simulink model "sm_robot_run_4legs"  (R2022b)
settings: Solver=ode15s  StartTime=0.0  StopTime=2  MaxStep=0.01  RelTol=1e-3  AbsTol=1e-4  EnableMultiTasking=on
InitFcn:
  | d2r = pi/180;
  | r2d = 180/pi;
  | if (~exist('t_final'))
  |   sm_robot_run_4legs_param_def_load(bdroot)
  | end
undefined symbols (not defined in the file): body_width, bw, Extr_Data_LinkEndHole, Extr_Data_Mesh, J, l1, L_back, L_stance, M, N, T_cg, t_th, t_w, th2, th2_0, Trq_propulsive, u0, u_th, u_w, X, Y, Z
libraries: sm_lib x60, fl_lib x57, nesl_utility x26, ee_lib x4, sm_robot_run_4legs_lib x4, batteryecm_lib x1
(part 4 of 4)

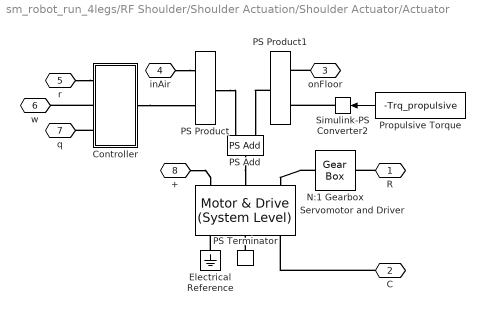
== system sm_robot_run_4legs/RF Shoulder/Shoulder Actuation/Shoulder Actuator/Actuator ==
  Controller : Subsystem
  Electrical Reference : fl_lib/Electrical/Electrical Elements/Electrical Reference
  N:1 Gearbox : fl_lib/Mechanical/Mechanisms/Gear Box  ratio=-N  t_in_specify=off  t_in_priority=None  t_in=0 N*m  t_in_nominal_specify=off  t_in_nominal_unit=N*m  t_in_nominal_value=1  t_out_specify=off  t_out_priority=None  t_out=0 N*m  t_out_nominal_specify=off  t_out_nominal_unit=N*m  t_out_nominal_value=1
  PS Add : fl_lib/Physical Signals/Functions/PS Add
  PS Product : fl_lib/Physical Signals/Functions/PS Product
  PS Product1 : fl_lib/Physical Signals/Functions/PS Product
  PS Terminator : fl_lib/Physical Signals/Sinks/PS Terminator
  Propulsive Torque : Constant  Value=-Trq_propulsive
  Servomotor and Driver : ee_lib/Electromechanical/Motor & Drive (System Level)  torque_speed_param=1  overtorque_param=ee.enum.electromech.overtorque.no  T_t="[  0.13 0.115 0.1 0 ]*5 N*m"  T_t_intermittent=[.36, .32, .28, 0] N*m  T_t_2D=[.09, .09, .09; .08, .08, .08; .07, .07, .07; 0, 0, 0] N*m  T_t_intermittent_2D=[.36, .36, .36; .32, .32, .32; .28, .28, .28; 0, 0, 0] N*m  w_t="[  0 2e+03 4e+03 4.1e3] rpm"  vdc_t=[6, 12, 24] V  torque_max=0.1 N*m  power_max=30 W  torque_max_intermittent=0.4 N*m  power_max_intermittent=120 W  time_overtorque=30 s  time_recover=60 s  Tc=0.01 s  losses_param=1  eff=100  w_eff=3.75e+3 rpm  T_eff=0.08 N*m  Piron=0 W  Pbase=0 W  w_eff_vec=[-8000 -4000 0 4000 8000] rpm  T_eff_vec=[0 0.03 0.06 0.09] N*m  v_eff_vec=[100, 250, 400] V  losses_mat=[1.49 1.67 2.21 3.10; 0.42 0.69 1.14 2.03; 0.06 0.24 0.78 1.68; 0.42 0.69 1.14 2.03; 1.49 1.67 2.21 3.10] W  efficiency_mat=[95 95 95 95; 95 95 95 95; 95 95 95 95; 95 95 95 95; 95 95 95 95]  losses_mat_3D=ones(5, 4, 3) W  efficiency_mat_3D=95 * ones(5, 4, 3)  Res=0.1 Ohm  enable_fault=simscape.enum.onoff.off  fault_condition=1  fault_threshold=0.5  J=0 g*cm^2  lam=0 N*m/(rad/s)  speed0=th1_dot_0*N rad/s  faulted_specify=off  faulted_priority=None  faulted=0  faulted_nominal_specify=off  faulted_nominal_unit=1  faulted_nominal_value=1  torqueLimitContinuous_specify=off  torqueLimitContinuous_priority=None  torqueLimitContinuous=0 N*m  torqueLimitContinuous_nominal_specify=off  torqueLimitContinuous_nominal_unit=N*m  torqueLimitContinuous_nominal_value=1  alpha=3.93e-3 1/K  Tmeas=25 degC  Tmeas2=125 degC  losses_mat_T2=[1.49, 1.74, 2.49, 3.74; .42, .67, 1.42, 2.67; .06, .31, 1.06, 2.31; .42, .67, 1.42, 2.67; 1.49, 1.74, 2.49, 3.74] W  efficiency_mat_T2=[95, 95, 95, 95; 95, 95, 95, 95; 95, 95, 95, 95; 95, 95, 95, 95; 95, 95, 95, 95]  losses_mat_3D_T2=ones(5, 4, 3) W  efficiency_mat_3D_T2=95 * ones(5, 4, 3)  thermal_mass=100 J/K  initial_temperature=25 degC
  Simulink-PS Converter2 : nesl_utility/Simulink-PS Converter  PhysicalDomain=network_engine_domain  SubClassName=ps_input  LeftPortType=input  RightPortType=output  PseudoPeriodic=off  Frequencies=[]  NoiseDistribution=none  NoiseParameters=[]  Unit=N*m  AffineConversion=off  FilteringAndDerivatives=zero  SimscapeFilterOrder=1  InputFilterTimeConstant=0.005  UdotUserProvided=0
  R : PMIOPort  Side=Right
  C : PMIOPort  Port=2  Side=Left
  onFloor : PMIOPort  Port=3  Side=Left
  inAir : PMIOPort  Port=4  Side=Left
  r : PMIOPort  Port=5  Side=Left
  w : PMIOPort  Port=6  Side=Right
  q : PMIOPort  Port=7  Side=Right
  + : PMIOPort  Port=8  Side=Right
  wires:
  Propulsive Torque/1 -> Simulink-PS Converter2/1
  connections:
  Simulink-PS Converter2/RConn1 -- PS Product1/LConn2
  PS Product1/RConn1 -- PS Add/LConn2
  onFloor/RConn1 -- PS Product1/LConn1
  PS Product/RConn1 -- PS Add/LConn1
  PS Add/RConn1 -- Servomotor and Driver/LConn2
  Controller/LConn2 -- w/RConn1
  Controller/LConn3 -- q/RConn1
  r/RConn1 -- Controller/LConn1
  Controller/RConn1 -- PS Product/LConn1
  +/RConn1 -- Servomotor and Driver/LConn1
  Electrical Reference/LConn1 -- Servomotor and Driver/RConn1
  C/RConn1 -- Servomotor and Driver/RConn3
  R/RConn1 -- N:1 Gearbox/RConn1
  N:1 Gearbox/LConn1 -- Servomotor and Driver/LConn3
  PS Terminator/LConn1 -- Servomotor and Driver/RConn2
  inAir/RConn1 -- PS Product/LConn2

== system sm_robot_run_4legs/RF Shoulder/Shoulder Actuation/Shoulder Actuator/Air or Floor ==
  aerial : Inport
  Data Type Conversion : DataTypeConversion  OutDataTypeStr=double  SaturateOnIntegerOverflow=off  RndMeth=Floor
  On ground : Fcn  Expr=1-u
  Simulink-PS Converter : nesl_utility/Simulink-PS Converter  PhysicalDomain=network_engine_domain  SubClassName=ps_input  LeftPortType=input  RightPortType=output  PseudoPeriodic=off  Frequencies=[]  NoiseDistribution=none  NoiseParameters=[]  Unit=1  AffineConversion=off  FilteringAndDerivatives=zero  SimscapeFilterOrder=1  InputFilterTimeConstant=0.005  UdotUserProvided=0
  Simulink-PS Converter1 : nesl_utility/Simulink-PS Converter  PhysicalDomain=network_engine_domain  SubClassName=ps_input  LeftPortType=input  RightPortType=output  PseudoPeriodic=off  Frequencies=[]  NoiseDistribution=none  NoiseParameters=[]  Unit=1  AffineConversion=off  FilteringAndDerivatives=zero  SimscapeFilterOrder=1  InputFilterTimeConstant=0.005  UdotUserProvided=0
  onFloor : PMIOPort  Side=Right
  inAir : PMIOPort  Port=2  Side=Right
  wires:
  aerial/1 -> Data Type Conversion/1
  On ground/1 -> Simulink-PS Converter1/1
  Data Type Conversion/1 -> Simulink-PS Converter/1, On ground/1
  connections:
  Simulink-PS Converter1/RConn1 -- onFloor/RConn1
  Simulink-PS Converter/RConn1 -- inAir/RConn1

== system sm_robot_run_4legs/RF Shoulder/Shoulder Actuation/Shoulder Actuator/Rotational Simscape Intf ==
  Angular Velocity Source : fl_lib/Mechanical/Mechanical Sources/Ideal Angular Velocity Source
  Torque Sensor : fl_lib/Mechanical/Mechanical Sensors/Ideal Torque Sensor
  w : PMIOPort  Side=Right
  t : PMIOPort  Port=2  Side=Left
  R : PMIOPort  Port=3  Side=Right
  C : PMIOPort  Port=4  Side=Left
  connections:
  w/RConn1 -- Angular Velocity Source/RConn1
  t/RConn1 -- Torque Sensor/RConn2
  Torque Sensor/LConn1 -- Angular Velocity Source/RConn2
  R/RConn1 -- Angular Velocity Source/LConn1
  Torque Sensor/RConn1 -- C/RConn1

== system sm_robot_run_4legs/RF Shoulder/Shoulder Actuation/Shoulder Actuator/Trajectory Demand ==
  aerial : Inport
  t_aerial : Inport  Port=2
  Enabled Subsystem : Subsystem  TreatAsAtomicUnit=on
  Gain : Gain  Gain=d2r
  Simulink-PS Converter : nesl_utility/Simulink-PS Converter  PhysicalDomain=network_engine_domain  SubClassName=ps_input  LeftPortType=input  RightPortType=output  PseudoPeriodic=off  Frequencies=[]  NoiseDistribution=none  NoiseParameters=[]  Unit=rad  AffineConversion=off  FilteringAndDerivatives=zero  SimscapeFilterOrder=1  InputFilterTimeConstant=0.005  UdotUserProvided=0
  Terminator : Terminator
  Terminator1 : Terminator
  r : PMIOPort  Side=Right
  wires:
  Enabled Subsystem/3(angle_dot) -> Terminator1/1
  Enabled Subsystem/2(angle) -> Terminator/1
  t_aerial/1 -> Enabled Subsystem/1(t_aerial)
  Enabled Subsystem/1(r) -> Gain/1
  aerial/1 -> Enabled Subsystem/Enable
  Gain/1 -> Simulink-PS Converter/1
  connections:
  r/RConn1 -- Simulink-PS Converter/RConn1

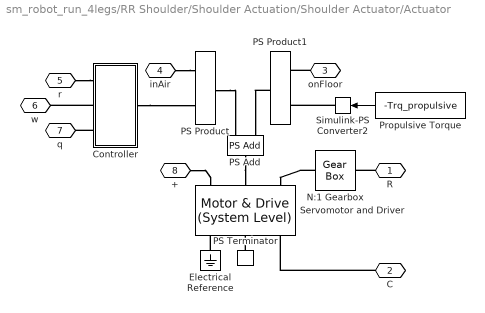
== system sm_robot_run_4legs/RR Shoulder/Shoulder Actuation/Shoulder Actuator/Actuator ==
  Controller : Subsystem
  Electrical Reference : fl_lib/Electrical/Electrical Elements/Electrical Reference
  N:1 Gearbox : fl_lib/Mechanical/Mechanisms/Gear Box  ratio=-N  t_in_specify=off  t_in_priority=None  t_in=0 N*m  t_in_nominal_specify=off  t_in_nominal_unit=N*m  t_in_nominal_value=1  t_out_specify=off  t_out_priority=None  t_out=0 N*m  t_out_nominal_specify=off  t_out_nominal_unit=N*m  t_out_nominal_value=1
  PS Add : fl_lib/Physical Signals/Functions/PS Add
  PS Product : fl_lib/Physical Signals/Functions/PS Product
  PS Product1 : fl_lib/Physical Signals/Functions/PS Product
  PS Terminator : fl_lib/Physical Signals/Sinks/PS Terminator
  Propulsive Torque : Constant  Value=-Trq_propulsive
  Servomotor and Driver : ee_lib/Electromechanical/Motor & Drive (System Level)  torque_speed_param=1  overtorque_param=ee.enum.electromech.overtorque.no  T_t="[  0.13 0.115 0.1 0 ]*5 N*m"  T_t_intermittent=[.36, .32, .28, 0] N*m  T_t_2D=[.09, .09, .09; .08, .08, .08; .07, .07, .07; 0, 0, 0] N*m  T_t_intermittent_2D=[.36, .36, .36; .32, .32, .32; .28, .28, .28; 0, 0, 0] N*m  w_t="[  0 2e+03 4e+03 4.1e3] rpm"  vdc_t=[6, 12, 24] V  torque_max=0.1 N*m  power_max=30 W  torque_max_intermittent=0.4 N*m  power_max_intermittent=120 W  time_overtorque=30 s  time_recover=60 s  Tc=0.01 s  losses_param=1  eff=100  w_eff=3.75e+3 rpm  T_eff=0.08 N*m  Piron=0 W  Pbase=0 W  w_eff_vec=[-8000 -4000 0 4000 8000] rpm  T_eff_vec=[0 0.03 0.06 0.09] N*m  v_eff_vec=[100, 250, 400] V  losses_mat=[1.49 1.67 2.21 3.10; 0.42 0.69 1.14 2.03; 0.06 0.24 0.78 1.68; 0.42 0.69 1.14 2.03; 1.49 1.67 2.21 3.10] W  efficiency_mat=[95 95 95 95; 95 95 95 95; 95 95 95 95; 95 95 95 95; 95 95 95 95]  losses_mat_3D=ones(5, 4, 3) W  efficiency_mat_3D=95 * ones(5, 4, 3)  Res=0.1 Ohm  enable_fault=simscape.enum.onoff.off  fault_condition=1  fault_threshold=0.5  J=0 g*cm^2  lam=0 N*m/(rad/s)  speed0=th1_dot_0*N rad/s  faulted_specify=off  faulted_priority=None  faulted=0  faulted_nominal_specify=off  faulted_nominal_unit=1  faulted_nominal_value=1  torqueLimitContinuous_specify=off  torqueLimitContinuous_priority=None  torqueLimitContinuous=0 N*m  torqueLimitContinuous_nominal_specify=off  torqueLimitContinuous_nominal_unit=N*m  torqueLimitContinuous_nominal_value=1  alpha=3.93e-3 1/K  Tmeas=25 degC  Tmeas2=125 degC  losses_mat_T2=[1.49, 1.74, 2.49, 3.74; .42, .67, 1.42, 2.67; .06, .31, 1.06, 2.31; .42, .67, 1.42, 2.67; 1.49, 1.74, 2.49, 3.74] W  efficiency_mat_T2=[95, 95, 95, 95; 95, 95, 95, 95; 95, 95, 95, 95; 95, 95, 95, 95; 95, 95, 95, 95]  losses_mat_3D_T2=ones(5, 4, 3) W  efficiency_mat_3D_T2=95 * ones(5, 4, 3)  thermal_mass=100 J/K  initial_temperature=25 degC
  Simulink-PS Converter2 : nesl_utility/Simulink-PS Converter  PhysicalDomain=network_engine_domain  SubClassName=ps_input  LeftPortType=input  RightPortType=output  PseudoPeriodic=off  Frequencies=[]  NoiseDistribution=none  NoiseParameters=[]  Unit=N*m  AffineConversion=off  FilteringAndDerivatives=zero  SimscapeFilterOrder=1  InputFilterTimeConstant=0.005  UdotUserProvided=0
  R : PMIOPort  Side=Right
  C : PMIOPort  Port=2  Side=Left
  onFloor : PMIOPort  Port=3  Side=Left
  inAir : PMIOPort  Port=4  Side=Left
  r : PMIOPort  Port=5  Side=Left
  w : PMIOPort  Port=6  Side=Right
  q : PMIOPort  Port=7  Side=Right
  + : PMIOPort  Port=8  Side=Right
  wires:
  Propulsive Torque/1 -> Simulink-PS Converter2/1
  connections:
  Simulink-PS Converter2/RConn1 -- PS Product1/LConn2
  PS Product1/RConn1 -- PS Add/LConn2
  onFloor/RConn1 -- PS Product1/LConn1
  PS Product/RConn1 -- PS Add/LConn1
  PS Add/RConn1 -- Servomotor and Driver/LConn2
  Controller/LConn2 -- w/RConn1
  Controller/LConn3 -- q/RConn1
  r/RConn1 -- Controller/LConn1
  Controller/RConn1 -- PS Product/LConn1
  +/RConn1 -- Servomotor and Driver/LConn1
  Electrical Reference/LConn1 -- Servomotor and Driver/RConn1
  C/RConn1 -- Servomotor and Driver/RConn3
  R/RConn1 -- N:1 Gearbox/RConn1
  N:1 Gearbox/LConn1 -- Servomotor and Driver/LConn3
  PS Terminator/LConn1 -- Servomotor and Driver/RConn2
  inAir/RConn1 -- PS Product/LConn2

== system sm_robot_run_4legs/RR Shoulder/Shoulder Actuation/Shoulder Actuator/Air or Floor ==
  aerial : Inport
  Data Type Conversion : DataTypeConversion  OutDataTypeStr=double  SaturateOnIntegerOverflow=off  RndMeth=Floor
  On ground : Fcn  Expr=1-u
  Simulink-PS Converter : nesl_utility/Simulink-PS Converter  PhysicalDomain=network_engine_domain  SubClassName=ps_input  LeftPortType=input  RightPortType=output  PseudoPeriodic=off  Frequencies=[]  NoiseDistribution=none  NoiseParameters=[]  Unit=1  AffineConversion=off  FilteringAndDerivatives=zero  SimscapeFilterOrder=1  InputFilterTimeConstant=0.005  UdotUserProvided=0
  Simulink-PS Converter1 : nesl_utility/Simulink-PS Converter  PhysicalDomain=network_engine_domain  SubClassName=ps_input  LeftPortType=input  RightPortType=output  PseudoPeriodic=off  Frequencies=[]  NoiseDistribution=none  NoiseParameters=[]  Unit=1  AffineConversion=off  FilteringAndDerivatives=zero  SimscapeFilterOrder=1  InputFilterTimeConstant=0.005  UdotUserProvided=0
  onFloor : PMIOPort  Side=Right
  inAir : PMIOPort  Port=2  Side=Right
  wires:
  aerial/1 -> Data Type Conversion/1
  On ground/1 -> Simulink-PS Converter1/1
  Data Type Conversion/1 -> Simulink-PS Converter/1, On ground/1
  connections:
  Simulink-PS Converter1/RConn1 -- onFloor/RConn1
  Simulink-PS Converter/RConn1 -- inAir/RConn1

== system sm_robot_run_4legs/RR Shoulder/Shoulder Actuation/Shoulder Actuator/Rotational Simscape Intf ==
  Angular Velocity Source : fl_lib/Mechanical/Mechanical Sources/Ideal Angular Velocity Source
  Torque Sensor : fl_lib/Mechanical/Mechanical Sensors/Ideal Torque Sensor
  w : PMIOPort  Side=Right
  t : PMIOPort  Port=2  Side=Left
  R : PMIOPort  Port=3  Side=Right
  C : PMIOPort  Port=4  Side=Left
  connections:
  w/RConn1 -- Angular Velocity Source/RConn1
  t/RConn1 -- Torque Sensor/RConn2
  Torque Sensor/LConn1 -- Angular Velocity Source/RConn2
  R/RConn1 -- Angular Velocity Source/LConn1
  Torque Sensor/RConn1 -- C/RConn1

== system sm_robot_run_4legs/RR Shoulder/Shoulder Actuation/Shoulder Actuator/Trajectory Demand ==
  aerial : Inport
  t_aerial : Inport  Port=2
  Enabled Subsystem : Subsystem  TreatAsAtomicUnit=on
  Gain : Gain  Gain=d2r
  Simulink-PS Converter : nesl_utility/Simulink-PS Converter  PhysicalDomain=network_engine_domain  SubClassName=ps_input  LeftPortType=input  RightPortType=output  PseudoPeriodic=off  Frequencies=[]  NoiseDistribution=none  NoiseParameters=[]  Unit=rad  AffineConversion=off  FilteringAndDerivatives=zero  SimscapeFilterOrder=1  InputFilterTimeConstant=0.005  UdotUserProvided=0
  Terminator : Terminator
  Terminator1 : Terminator
  r : PMIOPort  Side=Right
  wires:
  Enabled Subsystem/3(angle_dot) -> Terminator1/1
  Enabled Subsystem/2(angle) -> Terminator/1
  t_aerial/1 -> Enabled Subsystem/1(t_aerial)
  Enabled Subsystem/1(r) -> Gain/1
  aerial/1 -> Enabled Subsystem/Enable
  Gain/1 -> Simulink-PS Converter/1
  connections:
  r/RConn1 -- Simulink-PS Converter/RConn1

== system sm_robot_run_4legs/LF Shoulder/Shoulder Actuation/Shoulder Actuator/Actuator/Controller ==
  K=bw*J/N : fl_lib/Physical Signals/Functions/PS Gain  gain=bw*J/N (N*m)/rad
  PS Add : fl_lib/Physical Signals/Functions/PS Add
  PS Add1 : fl_lib/Physical Signals/Functions/PS Add
  PS Gain : fl_lib/Physical Signals/Functions/PS Gain  gain=0.1 s
  r : PMIOPort  Side=Left
  w : PMIOPort  Port=2  Side=Left
  T : PMIOPort  Port=3  Side=Right
  q : PMIOPort  Port=4  Side=Left
  connections:
  w/RConn1 -- PS Gain/LConn1
  PS Add1/RConn1 -- K=bw*J/N/LConn1
  T/RConn1 -- K=bw*J/N/RConn1
  PS Gain/RConn1 -- PS Add/LConn1
  PS Add1/LConn2 -- PS Add/RConn1
  q/RConn1 -- PS Add/LConn2
  PS Add1/LConn1 -- r/RConn1

== system sm_robot_run_4legs/LF Shoulder/Shoulder Actuation/Shoulder Actuator/Trajectory Demand/Enabled Subsystem ==
  t_aerial : Inport
  Enable : EnablePort  StatesWhenEnabling=reset
  Gain3 : Gain  Gain=0.1
  Lookup Table : Lookup  InputValues=t_th  Table=u_th  LookUpMeth=Interpolation-Use End Values  SaturateOnIntegerOverflow=off
  Lookup Table1 : Lookup  InputValues=t_w  Table=u_w  LookUpMeth=Interpolation-Use End Values  SaturateOnIntegerOverflow=off
  Sum : Sum  Inputs=|++
  r : Outport  OutputWhenDisabled=reset  InitialOutput=[0]  VectorParamsAs1DForOutWhenUnconnected=off
  angle : Outport  Port=2  OutputWhenDisabled=reset  InitialOutput=[0]  VectorParamsAs1DForOutWhenUnconnected=off
  angle_dot : Outport  Port=3  OutputWhenDisabled=reset  InitialOutput=[0]  VectorParamsAs1DForOutWhenUnconnected=off
  wires:
  Gain3/1 -> Sum/2
  Sum/1 -> r/1
  Lookup Table/1 -> Sum/1, angle/1
  t_aerial/1 -> Lookup Table1/1, Lookup Table/1
  Lookup Table1/1 -> Gain3/1, angle_dot/1

== system sm_robot_run_4legs/LR Shoulder/Shoulder Actuation/Shoulder Actuator/Actuator/Controller ==
  K=bw*J/N : fl_lib/Physical Signals/Functions/PS Gain  gain=bw*J/N (N*m)/rad
  PS Add : fl_lib/Physical Signals/Functions/PS Add
  PS Add1 : fl_lib/Physical Signals/Functions/PS Add
  PS Gain : fl_lib/Physical Signals/Functions/PS Gain  gain=0.1 s
  r : PMIOPort  Side=Left
  w : PMIOPort  Port=2  Side=Left
  T : PMIOPort  Port=3  Side=Right
  q : PMIOPort  Port=4  Side=Left
  connections:
  w/RConn1 -- PS Gain/LConn1
  PS Add1/RConn1 -- K=bw*J/N/LConn1
  T/RConn1 -- K=bw*J/N/RConn1
  PS Gain/RConn1 -- PS Add/LConn1
  PS Add1/LConn2 -- PS Add/RConn1
  q/RConn1 -- PS Add/LConn2
  PS Add1/LConn1 -- r/RConn1

== system sm_robot_run_4legs/LR Shoulder/Shoulder Actuation/Shoulder Actuator/Trajectory Demand/Enabled Subsystem ==
  t_aerial : Inport
  Enable : EnablePort  StatesWhenEnabling=reset
  Gain3 : Gain  Gain=0.1
  Lookup Table : Lookup  InputValues=t_th  Table=u_th  LookUpMeth=Interpolation-Use End Values  SaturateOnIntegerOverflow=off
  Lookup Table1 : Lookup  InputValues=t_w  Table=u_w  LookUpMeth=Interpolation-Use End Values  SaturateOnIntegerOverflow=off
  Sum : Sum  Inputs=|++
  r : Outport  OutputWhenDisabled=reset  InitialOutput=[0]  VectorParamsAs1DForOutWhenUnconnected=off
  angle : Outport  Port=2  OutputWhenDisabled=reset  InitialOutput=[0]  VectorParamsAs1DForOutWhenUnconnected=off
  angle_dot : Outport  Port=3  OutputWhenDisabled=reset  InitialOutput=[0]  VectorParamsAs1DForOutWhenUnconnected=off
  wires:
  Gain3/1 -> Sum/2
  Sum/1 -> r/1
  Lookup Table/1 -> Sum/1, angle/1
  t_aerial/1 -> Lookup Table1/1, Lookup Table/1
  Lookup Table1/1 -> Gain3/1, angle_dot/1

== system sm_robot_run_4legs/RF Shoulder/Shoulder Actuation/Shoulder Actuator/Actuator/Controller ==
  K=bw*J/N : fl_lib/Physical Signals/Functions/PS Gain  gain=bw*J/N (N*m)/rad
  PS Add : fl_lib/Physical Signals/Functions/PS Add
  PS Add1 : fl_lib/Physical Signals/Functions/PS Add
  PS Gain : fl_lib/Physical Signals/Functions/PS Gain  gain=0.1 s
  r : PMIOPort  Side=Left
  w : PMIOPort  Port=2  Side=Left
  T : PMIOPort  Port=3  Side=Right
  q : PMIOPort  Port=4  Side=Left
  connections:
  w/RConn1 -- PS Gain/LConn1
  PS Add1/RConn1 -- K=bw*J/N/LConn1
  T/RConn1 -- K=bw*J/N/RConn1
  PS Gain/RConn1 -- PS Add/LConn1
  PS Add1/LConn2 -- PS Add/RConn1
  q/RConn1 -- PS Add/LConn2
  PS Add1/LConn1 -- r/RConn1

== system sm_robot_run_4legs/RF Shoulder/Shoulder Actuation/Shoulder Actuator/Trajectory Demand/Enabled Subsystem ==
  t_aerial : Inport
  Enable : EnablePort  StatesWhenEnabling=reset
  Gain3 : Gain  Gain=0.1
  Lookup Table : Lookup  InputValues=t_th  Table=u_th  LookUpMeth=Interpolation-Use End Values  SaturateOnIntegerOverflow=off
  Lookup Table1 : Lookup  InputValues=t_w  Table=u_w  LookUpMeth=Interpolation-Use End Values  SaturateOnIntegerOverflow=off
  Sum : Sum  Inputs=|++
  r : Outport  OutputWhenDisabled=reset  InitialOutput=[0]  VectorParamsAs1DForOutWhenUnconnected=off
  angle : Outport  Port=2  OutputWhenDisabled=reset  InitialOutput=[0]  VectorParamsAs1DForOutWhenUnconnected=off
  angle_dot : Outport  Port=3  OutputWhenDisabled=reset  InitialOutput=[0]  VectorParamsAs1DForOutWhenUnconnected=off
  wires:
  Gain3/1 -> Sum/2
  Sum/1 -> r/1
  Lookup Table/1 -> Sum/1, angle/1
  t_aerial/1 -> Lookup Table1/1, Lookup Table/1
  Lookup Table1/1 -> Gain3/1, angle_dot/1

== system sm_robot_run_4legs/RR Shoulder/Shoulder Actuation/Shoulder Actuator/Actuator/Controller ==
  K=bw*J/N : fl_lib/Physical Signals/Functions/PS Gain  gain=bw*J/N (N*m)/rad
  PS Add : fl_lib/Physical Signals/Functions/PS Add
  PS Add1 : fl_lib/Physical Signals/Functions/PS Add
  PS Gain : fl_lib/Physical Signals/Functions/PS Gain  gain=0.1 s
  r : PMIOPort  Side=Left
  w : PMIOPort  Port=2  Side=Left
  T : PMIOPort  Port=3  Side=Right
  q : PMIOPort  Port=4  Side=Left
  connections:
  w/RConn1 -- PS Gain/LConn1
  PS Add1/RConn1 -- K=bw*J/N/LConn1
  T/RConn1 -- K=bw*J/N/RConn1
  PS Gain/RConn1 -- PS Add/LConn1
  PS Add1/LConn2 -- PS Add/RConn1
  q/RConn1 -- PS Add/LConn2
  PS Add1/LConn1 -- r/RConn1

== system sm_robot_run_4legs/RR Shoulder/Shoulder Actuation/Shoulder Actuator/Trajectory Demand/Enabled Subsystem ==
  t_aerial : Inport
  Enable : EnablePort  StatesWhenEnabling=reset
  Gain3 : Gain  Gain=0.1
  Lookup Table : Lookup  InputValues=t_th  Table=u_th  LookUpMeth=Interpolation-Use End Values  SaturateOnIntegerOverflow=off
  Lookup Table1 : Lookup  InputValues=t_w  Table=u_w  LookUpMeth=Interpolation-Use End Values  SaturateOnIntegerOverflow=off
  Sum : Sum  Inputs=|++
  r : Outport  OutputWhenDisabled=reset  InitialOutput=[0]  VectorParamsAs1DForOutWhenUnconnected=off
  angle : Outport  Port=2  OutputWhenDisabled=reset  InitialOutput=[0]  VectorParamsAs1DForOutWhenUnconnected=off
  angle_dot : Outport  Port=3  OutputWhenDisabled=reset  InitialOutput=[0]  VectorParamsAs1DForOutWhenUnconnected=off
  wires:
  Gain3/1 -> Sum/2
  Sum/1 -> r/1
  Lookup Table/1 -> Sum/1, angle/1
  t_aerial/1 -> Lookup Table1/1, Lookup Table/1
  Lookup Table1/1 -> Gain3/1, angle_dot/1

== stateflow chart sm_robot_run_4legs/Gait Phase ==
  state Phase2
    entry: phase = 2;
    RL_FR_aerial =1;
  state Phase1
    entry: phase = 1;
  state Phase3
    entry: phase = 3;
  state Phase4
    entry: phase = 4;
    RR_FL_aerial=0;
  state Phase6
    entry: phase = 6;
    RR_FL_aerial=1;
  state Phase8
    entry: phase = 8;
    RL_FR_aerial=0;
  state Phase7
    entry: phase = 7;
  state Phase5
    entry: phase = 5;
  Phase1 -> Phase2 : [FR_flr==0]
  Phase2 -> Phase3 : [hdot<0]
  Phase3 -> Phase4 : [FL_flr==1]
  (junction 41) -> Phase1 : {RR_FL_aerial=1;}
  Phase8 -> Phase1
  Phase4 -> Phase5
  (default) -> (junction 41)
  Phase5 -> Phase6 : [FL_flr==0]
  Phase6 -> Phase7 : [hdot<0]
  Phase7 -> Phase8 : [FR_flr==1]
  data: FL_flr input; FR_flr input; hdot input; RL_FR_aerial output double; RR_FL_aerial output double; phase output double
